simulink model "NL_System"  (R2020a)
settings: Solver=ode4  StartTime=0.0  StopTime=10.0  RelTol=1e-3
values from neighbouring files (symbols this model uses):
  A = [0 0 0 1 0 0 ... (first row only)    [Aircraft_parameters.m]
  B = [0 0 ... (first row only)    [Aircraft_parameters.m]
  C = eye(3,6)    [Aircraft_parameters.m]
  L = place(A', C', pl)'    [main.m]
  Params = [g c m j r]    [Aircraft_parameters.m]
  use_output = 0    [main.m]
  use_state = 1    [main.m]
  x_inital = x0-x_bar    [Aircraft_parameters.m]
undefined symbols (not defined in the file or in its folder): K
settings Model: Creator=james  LastModifiedBy=connor

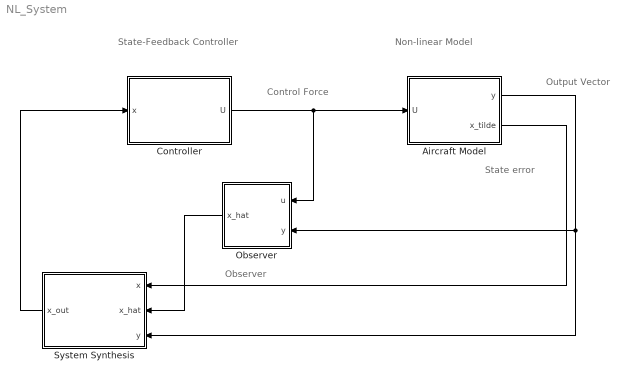
== system NL_System ==
  note: Control Force
  note: State-Feedback
      | Controller
  note: Non-linear Model
  note: Output Vector
  note: Observer
  note: State error
  "Aircraft Model " : Subsystem
  Controller : Subsystem
  Observer : Subsystem
  System Synthesis : Subsystem
  wires:
  Controller/1(U) -> Observer/1(u), "Aircraft Model "/1(U)
  "Aircraft Model "/1(y) -> Observer/2(y), System Synthesis/3(y)
  "Aircraft Model "/2(x_tilde) -> System Synthesis/1(x)
  System Synthesis/1(x_out) -> Controller/1(x)
  Observer/1(x_hat) -> System Synthesis/2(x_hat)

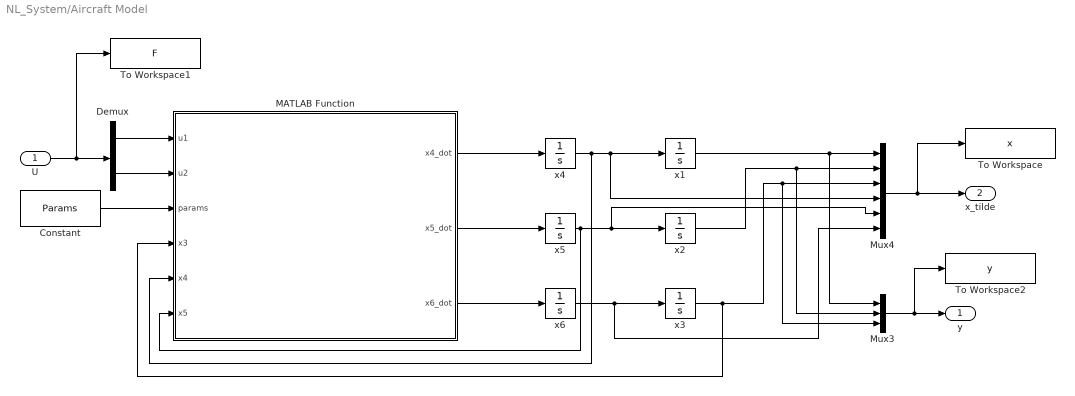
== system NL_System/Aircraft Model  ==
  U : Inport
  Constant : Constant  Value=Params
  Demux : Demux  Outputs=2
  MATLAB Function : MATLAB Function  TreatAsAtomicUnit=on
  Mux3 : Mux  Inputs=3
  Mux4 : Mux  Inputs=6
  To Workspace : ToWorkspace  VariableName=x  SampleTime=-1
  To Workspace1 : ToWorkspace  VariableName=F  SampleTime=-1
  To Workspace2 : ToWorkspace  VariableName=y  SampleTime=-1
  x1 : Integrator  InitialCondition=x_inital(1)
  x2 : Integrator  InitialCondition=x_inital(2)
  x3 : Integrator  InitialCondition=x_inital(3)
  x4 : Integrator  InitialCondition=x_inital(4)
  x5 : Integrator  InitialCondition=x_inital(5)
  x6 : Integrator  InitialCondition=x_inital(6)
  y : Outport
  x_tilde : Outport  Port=2
  wires:
  U/1 -> To Workspace1/1, Demux/1
  Constant/1 -> MATLAB Function/3(params)
  Demux/1 -> MATLAB Function/1(u1)
  Demux/2 -> MATLAB Function/2(u2)
  MATLAB Function/1(x4_dot) -> x4/1
  x4/1 -> MATLAB Function/5(x4), Mux4/4, x1/1
  MATLAB Function/2(x5_dot) -> x5/1
  MATLAB Function/3(x6_dot) -> x6/1
  x6/1 -> Mux4/6, x3/1
  x5/1 -> MATLAB Function/6(x5), Mux4/5, x2/1
  Mux3/1 -> To Workspace2/1, y/1
  Mux4/1 -> To Workspace/1, x_tilde/1
  x1/1 -> Mux3/1, Mux4/1
  x2/1 -> Mux3/2, Mux4/2
  x3/1 -> MATLAB Function/4(x3), Mux3/3, Mux4/3

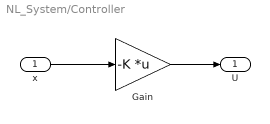
== system NL_System/Controller ==
  x : Inport
  Gain : Gain  Gain=-K  Multiplication=Matrix(K*u)
  U : Outport
  wires:
  x/1 -> Gain/1
  Gain/1 -> U/1

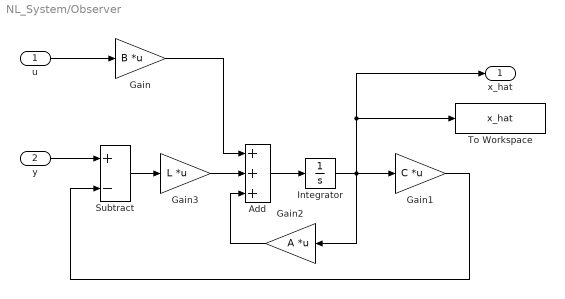
== system NL_System/Observer ==
  u : Inport
  y : Inport  Port=2
  Add : Sum  Inputs=3
  Gain : Gain  Gain=B  Multiplication=Matrix(K*u)
  Gain1 : Gain  Gain=C  Multiplication=Matrix(K*u)
  Gain2 : Gain  Gain=A  Multiplication=Matrix(K*u)
  Gain3 : Gain  Gain=L  Multiplication=Matrix(K*u)
  Integrator : Integrator
  Subtract : Sum  Inputs=+-
  To Workspace : ToWorkspace  VariableName=x_hat  SampleTime=-1
  x_hat : Outport
  wires:
  y/1 -> Subtract/1
  u/1 -> Gain/1
  Gain/1 -> Add/1
  Gain1/1 -> Subtract/2
  Gain2/1 -> Add/3
  Add/1 -> Integrator/1
  Integrator/1 -> Gain2/1, To Workspace/1, x_hat/1, Gain1/1
  Gain3/1 -> Add/2
  Subtract/1 -> Gain3/1

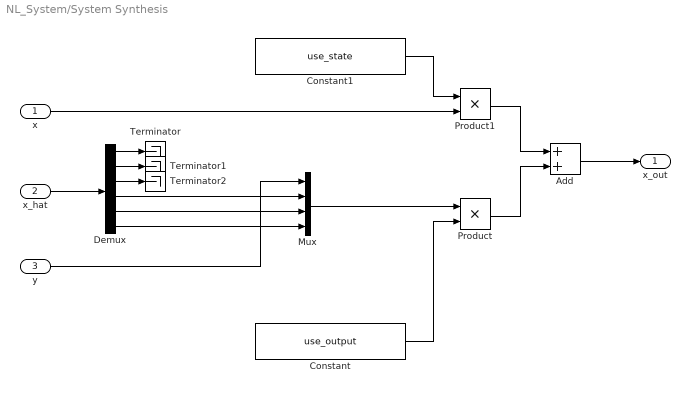
== system NL_System/System Synthesis ==
  x : Inport
  x_hat : Inport  Port=2
  y : Inport  Port=3
  Add : Sum
  Constant : Constant  Value=use_output
  Constant1 : Constant  Value=use_state
  Demux : Demux  Outputs=6
  Mux : Mux
  Product : Product
  Product1 : Product
  Terminator : Terminator
  Terminator1 : Terminator
  Terminator2 : Terminator
  x_out : Outport
  wires:
  Constant/1 -> Product/2
  Constant1/1 -> Product1/1
  x/1 -> Product1/2
  Product1/1 -> Add/1
  Add/1 -> x_out/1
  Product/1 -> Add/2
  x_hat/1 -> Demux/1
  Demux/6 -> Mux/4
  y/1 -> Mux/1
  Mux/1 -> Product/1
  Demux/1 -> Terminator/1
  Demux/2 -> Terminator1/1
  Demux/3 -> Terminator2/1
  Demux/5 -> Mux/3
  Demux/4 -> Mux/2

== matlab function NL_System/Aircraft Model /MATLAB Function ==
  data: u1 input; x4_dot output; u2 input; params input; x3 input; x4 input; x5 input; x5_dot output; x6_dot output
function [x4_dot, x5_dot, x6_dot] = NonLinearEquations(u1, u2, params, x3, x4, x5)

g = params(1);
c = params(2);
m = params(3);
j = params(4);
r = params(5);

x4_dot = ((-m*g*sin(x3))-(c*x4)+(u1*cos(x3))-(u2*sin(x3)))/m;
x5_dot = (((m*g)*((cos(x3)-1))) - (c*x5) + (u1*sin(x3))+(u2*cos(x3)))/m; 
x6_dot = (r*u1)/j;
